simulink model "trajStab"  (R2016b)
settings: Solver=FixedStepAuto  StartTime=0.0  StopTime=12  FixedStep=prms.Ts  RelTol=1e-3
PreLoadFcn:
  | Ts = 1e-3
undefined symbols (not defined in the file or in its folder): DiscIntNeverNeededParam, H, P0, prms, x0
libraries: simulink x1
PreSaveFcn:
  | set_param(gcs, 'location', [15 50 815 560])
settings Model: SimulationMode=external  Creator=The MathWorks Inc.  LastModifiedBy=marti
settings SolverCC: PositivePriorityOrder=on
settings DataIOCC: LimitDataPoints=on  SaveFormat=Array
settings OptimizationCC: BlockReduction=off  BooleanDataType=off  DefaultUnderspecifiedDataType=single  LifeSpan=inf  MaxStackSize=64
settings DebuggingCC: SaveWithParameterizedLinksMsg=none  UnderspecifiedInitializationDetection=Classic  MergeDetectMultiDrivingBlocksExec=none  SignalResolutionControl=TryResolveAllWithWarning  ParameterTunabilityLossMsg=error  SFUnexpectedBacktrackingDiag=warning  SFNoUnconditionalDefaultTransitionDiag=warning  SFExecutionAtInitializationDiag=none
settings HardwareCC: ProdBitPerPointer=32  ProdBitPerSizeT=32  ProdBitPerPtrDiffT=32  ProdLargestAtomicInteger=Long  ProdLargestAtomicFloat=Double  ProdWordSize=32  ProdHWDeviceType=ARM Compatible->ARM Cortex
settings ModelReferenceCC: PropagateSignalLabelsOutOfModel=off
settings RTWCC: SystemTargetFile=ert.tlc  HardwareBoard=Raspberry Pi  TLCOptions=-aInlineSetEventsForThisBaseRateFcn=TLC_FALSE -aSuppressMultiTaskScheduler=TLC_FALSE -aRateBasedStepFcn=0  TemplateMakefile=ert_default_tmf  Description=Embedded Coder  GenerateReport=on  RTWVerbose=off  Toolchain=GNU GCC Raspberry Pi  BuildConfiguration=Specify  IncludeHyperlinkInReport=on  GenerateTraceInfo=on  GenerateTraceReport=on  GenerateTraceReportSl=on  GenerateTraceReportSf=on  GenerateTraceReportEml=on
settings CodeAppCC: ForceParamTrailComments=on  IgnoreCustomStorageClasses=off  OperatorAnnotations=on  SimulinkDataObjDesc=on  SFDataObjDesc=on  MATLABFcnDesc=on  MangleLength=10  InsertBlockDesc=on  MATLABSourceComments=on
settings ERTTargetCC: SupportVariableSizeSignals=on
settings ConfigComp: CovMetricSettings=dw  CovHtmlReporting=on  CovSaveCumulativeToWorkspaceVar=on  CovSaveSingleToWorkspaceVar=on  CovExternalEMLEnable=off  CovSFcnEnable=off

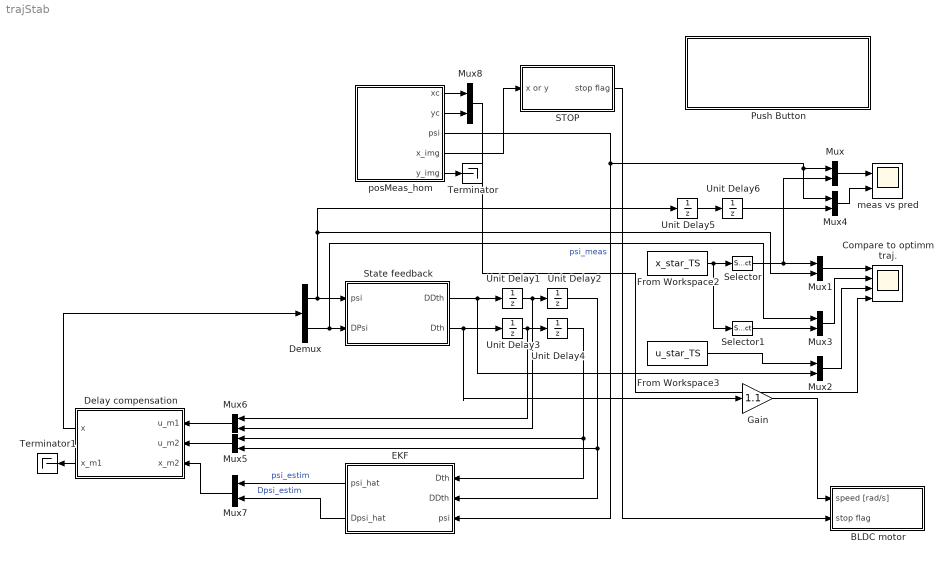
== system trajStab ==
  BLDC motor : Subsystem
  Compare to optimm traj. : Scope  NumInputPorts=4
  Delay compensation : Subsystem
  Demux : Demux  Outputs=2
  EKF : Subsystem
  From Workspace2 : FromWorkspace  VariableName=x_star_TS  OutDataTypeStr=single  SampleTime=prms.Ts  Interpolate=off  OutputAfterFinalValue=Setting to zero
  From Workspace3 : FromWorkspace  VariableName=u_star_TS  SampleTime=prms.Ts  Interpolate=off  OutputAfterFinalValue=Setting to zero
  Gain : Gain  Gain=1.1
  Mux{,1..8} (9 alike) : Mux  Inputs=2
  Push Button : Subsystem  DialogController=hmiCreateDDGDialog  IsWebBlock=on  mask(MWDashboardBlock){webBlockId=aa30e358-d2c6-466c-a89a-de069679829e, webBlockType=pushbutton, ShowInLibBrwoser=on, ShowInitialText=on, HMISrcModelName=trajStab}
      mask prompts: webBlockId "WebBlock Id"; webBlockType "WebBlock Type"; HMISrcModelName "Source Model"
      mask help: SimulinkHMI:dialogs:PushButtonDialogDesc
      mask Help: helpview([docroot '/mapfiles/simulink.map'], 'hmi_push_button')
      mask Display:
      | model = bdroot(gcb);
      | if strcmp(get_param(model,'BlockDiagramType'), 'library')
      |     image([(matlabroot) '/toolbox/simulink/hmi/icons/PushButton.png']);
      | end
  STOP : Subsystem
  Selector : Selector  InputPortWidth=3  IndexOptions=Index vector (dialog)  Indices=2  OutputSizes=1
  Selector1 : Selector  InputPortWidth=3  IndexOptions=Index vector (dialog)  Indices=3  OutputSizes=1
  State feedback : Subsystem
  Terminator : Terminator
  Terminator1 : Terminator
  Unit Delay{1..6} (6 alike) : UnitDelay  SampleTime=-1
  meas vs pred : Scope  NumInputPorts=2
  posMeas_hom : Subsystem
  wires:
  posMeas_hom/3(psi) -> EKF/3(psi), Mux4/1, Mux/1  "psi_meas"
  Mux/1 -> meas vs pred/1
  Mux1/1 -> Compare to optimm traj./1
  From Workspace3/1 -> Mux2/1
  From Workspace2/1 -> Selector1/1, Selector/1
  Selector/1 -> Mux1/1, Mux/2
  State feedback/2(Dth) -> Gain/1, Unit Delay3/1
  Unit Delay1/1 -> Mux6/2, Unit Delay2/1
  Mux5/1 -> Delay compensation/2(u_m2)
  Mux6/1 -> Delay compensation/1(u_m1)
  EKF/2(Dpsi_hat) -> Mux7/2  "Dpsi_estim"
  EKF/1(psi_hat) -> Mux7/1  "psi_estim"
  Unit Delay2/1 -> EKF/2(DDth), Mux5/2
  Unit Delay4/1 -> Mux5/1, EKF/1(Dth)
  Unit Delay3/1 -> Mux6/1, Unit Delay4/1
  Delay compensation/1(x) -> Demux/1
  Demux/2 -> Mux3/1, State feedback/2(DPsi)
  State feedback/1(DDth) -> Unit Delay1/1, Mux2/2
  Demux/1 -> State feedback/1(psi), Mux1/2, Unit Delay5/1
  Mux7/1 -> Delay compensation/3(x_m2)
  Mux3/1 -> Compare to optimm traj./2
  Mux2/1 -> Compare to optimm traj./3
  Selector1/1 -> Mux3/2
  STOP/1(stop flag) -> BLDC motor/2(stop flag)
  Mux4/1 -> meas vs pred/2
  Unit Delay6/1 -> Mux4/2
  Unit Delay5/1 -> Unit Delay6/1
  Delay compensation/2(x_m1) -> Terminator1/1
  posMeas_hom/5(y_img) -> Terminator/1
  posMeas_hom/4(x_img) -> STOP/1(x or y)
  posMeas_hom/1(xc) -> Mux8/1
  posMeas_hom/2(yc) -> Mux8/2
  Mux8/1 -> Compare to optimm traj./4
  Gain/1 -> BLDC motor/1(speed [rad/s])

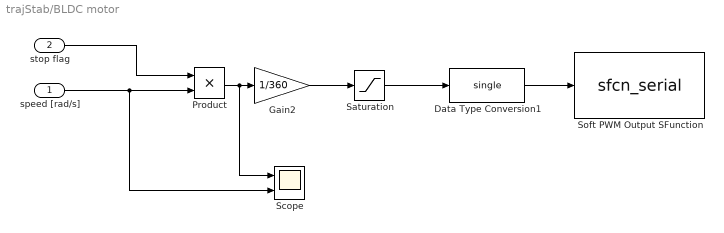
== system trajStab/BLDC motor ==
  speed [rad/s] : Inport
  stop flag : Inport  Port=2
  Data Type Conversion1 : DataTypeConversion  OutDataTypeStr=single
  Gain2 : Gain  Gain=1/360
  Product : Product
  Saturation : Saturate  UpperLimit=0.3  LowerLimit=-0.3
  Scope : Scope  NumInputPorts=2
  Soft PWM Output SFunction : S-Function  InitFcn=try, set_param(gcb,'FunctionName','sfcn_serial'), end  FunctionName=sfcn_serial  SFunctionModules=sfcn_serial_wrapper  SFunctionDeploymentMode=off  EnableBusSupport=off  mask(S-Function Builder){}
      mask init:
      | val = [[.9  0.75 0.75 1 1 .9 .9 1]',[1 1 0.75 0.75 .9 .9 1 .9]'];try , sys = get_param(gcb,'SfunBuilderFcnName');if isempty(sys), sys = get_param(gcb,'FunctionName'); end,catch, sys = get_param(gcb,'FunctionName'); end
      settings: CopyFcn=set_param(gcbh,'LinkStatus','none')  PreSaveFcn=try, set_param(gcb,'FunctionName','sfcn_serial'), end  OpenFcn=sfunctionwizard(gcbh)
      mask Display: plot(val(:,1),val(:,2)),disp(sys), port_label('input',1,'in')
  wires:
  Saturation/1 -> Data Type Conversion1/1
  Gain2/1 -> Saturation/1
  Data Type Conversion1/1 -> Soft PWM Output SFunction/1
  Product/1 -> Scope/1, Gain2/1
  speed [rad/s]/1 -> Scope/2, Product/2
  stop flag/1 -> Product/1

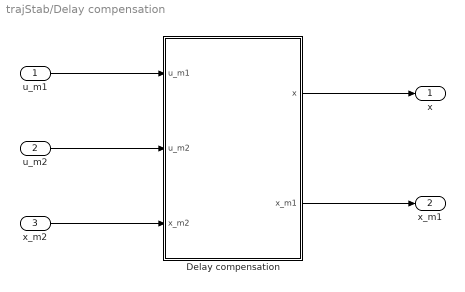
== system trajStab/Delay compensation ==
  u_m1 : Inport
  u_m2 : Inport  Port=2
  x_m2 : Inport  Port=3
  Delay compensation : MATLAB Function  TreatAsAtomicUnit=on  SystemSampleTime=prms.Ts
  x : Outport
  x_m1 : Outport  Port=2
  wires:
  x_m2/1 -> Delay compensation/3(x_m2)
  u_m1/1 -> Delay compensation/1(u_m1)
  u_m2/1 -> Delay compensation/2(u_m2)
  Delay compensation/1(x) -> x/1
  Delay compensation/2(x_m1) -> x_m1/1

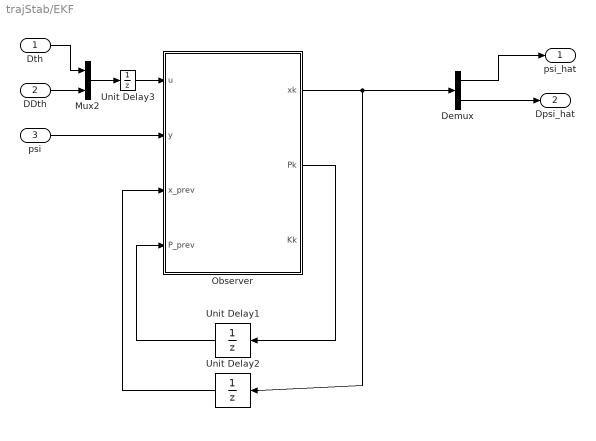
== system trajStab/EKF ==
  Dth : Inport
  DDth : Inport  Port=2
  psi : Inport  Port=3
  Demux : Demux  Outputs=2
  Mux2 : Mux  Inputs=2
  Observer : MATLAB Function  TreatAsAtomicUnit=on  SystemSampleTime=prms.Ts
  Unit Delay1 : UnitDelay  InitialCondition=P0  SampleTime=-1
  Unit Delay2 : UnitDelay  InitialCondition=x0  SampleTime=-1
  Unit Delay3 : UnitDelay  SampleTime=-1
  psi_hat : Outport
  Dpsi_hat : Outport  Port=2
  wires:
  Unit Delay2/1 -> Observer/3(x_prev)
  Observer/2(Pk) -> Unit Delay1/1
  Unit Delay1/1 -> Observer/4(P_prev)
  Observer/1(xk) -> Demux/1, Unit Delay2/1
  Demux/2 -> Dpsi_hat/1
  Demux/1 -> psi_hat/1
  Mux2/1 -> Unit Delay3/1
  Dth/1 -> Mux2/1
  DDth/1 -> Mux2/2
  psi/1 -> Observer/2(y)
  Unit Delay3/1 -> Observer/1(u)

== system trajStab/Push Button ==

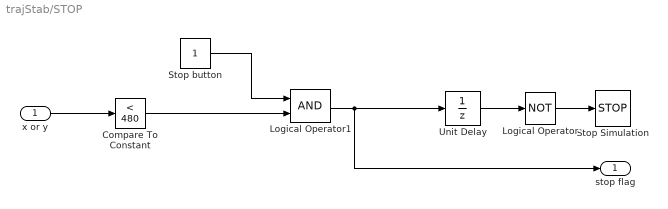
== system trajStab/STOP ==
  x or y : Inport
  Compare To Constant : simulink/Logic and Bit Operations/Compare To Constant  relop=<  const=480  OutDataTypeStr=boolean
  Logical Operator : Logic  Operator=NOT  AllPortsSameDT=off  OutDataTypeStr=boolean
  Logical Operator1 : Logic  AllPortsSameDT=off  OutDataTypeStr=boolean
  Stop Simulation : Stop
  Stop button : Constant
  Unit Delay : UnitDelay  InitialCondition=1  SampleTime=-1
  stop flag : Outport
  wires:
  Logical Operator/1 -> Stop Simulation/1
  Logical Operator1/1 -> stop flag/1, Unit Delay/1
  Unit Delay/1 -> Logical Operator/1
  Compare To Constant/1 -> Logical Operator1/2
  Stop button/1 -> Logical Operator1/1
  x or y/1 -> Compare To Constant/1

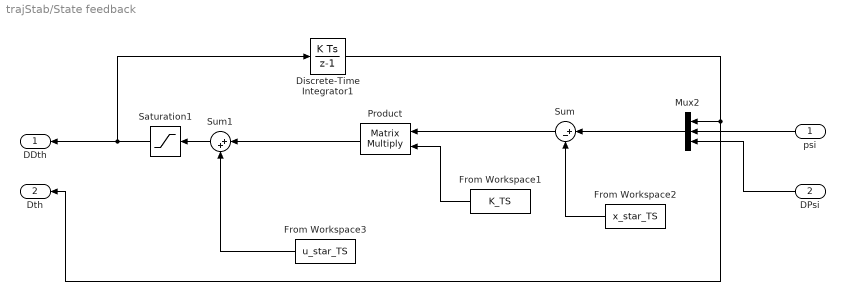
== system trajStab/State feedback ==
  psi : Inport
  DPsi : Inport  Port=2
  Discrete-Time Integrator1 : DiscreteIntegrator  InitialConditionSetting=State (most efficient)  SampleTime=prms.Ts  ICPrevOutput=DiscIntNeverNeededParam  ICPrevScaledInput=DiscIntNeverNeededParam
  From Workspace1 : FromWorkspace  VariableName=K_TS  OutDataTypeStr=single  SampleTime=prms.Ts  Interpolate=off  OutputAfterFinalValue=Setting to zero
  From Workspace2 : FromWorkspace  VariableName=x_star_TS  OutDataTypeStr=single  SampleTime=prms.Ts  Interpolate=off  OutputAfterFinalValue=Setting to zero
  From Workspace3 : FromWorkspace  VariableName=u_star_TS  OutDataTypeStr=single  SampleTime=prms.Ts  Interpolate=off  OutputAfterFinalValue=Setting to zero
  Mux2 : Mux  Inputs=3
  Product : Product  Multiplication=Matrix(*)
  Saturation1 : Saturate  UpperLimit=prms.usat  LowerLimit=-prms.usat
  Sum : Sum  Inputs=|+-
  Sum1 : Sum  Inputs=|++
  DDth : Outport
  Dth : Outport  Port=2
  wires:
  From Workspace1/1 -> Product/2
  Mux2/1 -> Sum/1
  From Workspace2/1 -> Sum/2
  Sum/1 -> Product/1
  From Workspace3/1 -> Sum1/2
  Sum1/1 -> Saturation1/1
  Saturation1/1 -> Discrete-Time Integrator1/1, DDth/1
  Discrete-Time Integrator1/1 -> Dth/1, Mux2/1
  psi/1 -> Mux2/2
  DPsi/1 -> Mux2/3
  Product/1 -> Sum1/1

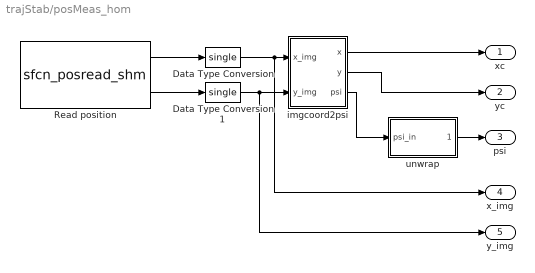
== system trajStab/posMeas_hom ==
  Data Type Conversion : DataTypeConversion  OutDataTypeStr=single
  Data Type Conversion1 : DataTypeConversion  OutDataTypeStr=single
  Read position : S-Function  InitFcn=try, set_param(gcb,'FunctionName','sfcn_posread_shm'), end  FunctionName=sfcn_posread_shm  SFunctionModules=sfcn_posread_shm_wrapper  SFunctionDeploymentMode=off  EnableBusSupport=off  mask(S-Function Builder){}
      mask init: same as trajStab/BLDC motor/Soft PWM Output SFunction
      settings: CopyFcn=set_param(gcbh,'LinkStatus','none')  PreSaveFcn=try, set_param(gcb,'FunctionName','sfcn_posread_shm'), end  OpenFcn=sfunctionwizard(gcbh)
      mask Display: plot(val(:,1),val(:,2)),disp(sys), port_label('output',1,'pos_x'), port_label('output',2,'pos_y')
  imgcoord2psi : Subsystem
  unwrap : Subsystem
  xc : Outport
  yc : Outport  Port=2
  psi : Outport  Port=3
  x_img : Outport  Port=4
  y_img : Outport  Port=5
  wires:
  Read position/1 -> Data Type Conversion/1
  Data Type Conversion/1 -> x_img/1, imgcoord2psi/1(x_img)
  Data Type Conversion1/1 -> y_img/1, imgcoord2psi/2(y_img)
  Read position/2 -> Data Type Conversion1/1
  imgcoord2psi/3(psi) -> unwrap/1(psi_in)
  unwrap/1(psi_out) -> psi/1
  imgcoord2psi/1(x) -> xc/1
  imgcoord2psi/2(y) -> yc/1

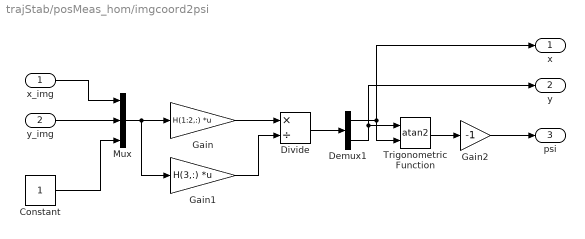
== system trajStab/posMeas_hom/imgcoord2psi ==
  x_img : Inport
  y_img : Inport  Port=2
  Constant : Constant  OutDataTypeStr=single
  Demux1 : Demux  Outputs=2
  Divide : Product  Inputs=*/
  Gain : Gain  Gain=H(1:2,:)  Multiplication=Matrix(K*u)
  Gain1 : Gain  Gain=H(3,:)  Multiplication=Matrix(K*u)
  Gain2 : Gain  Gain=-1  OutDataTypeStr=single
  Mux : Mux  Inputs=3
  Trigonometric Function : Trigonometry  Operator=atan2  OutputSignalType=real
  x : Outport
  y : Outport  Port=2
  psi : Outport  Port=3
  wires:
  Mux/1 -> Gain1/1, Gain/1
  Constant/1 -> Mux/3
  Demux1/2 -> y/1, Trigonometric Function/1
  Gain/1 -> Divide/1
  Gain1/1 -> Divide/2
  Divide/1 -> Demux1/1
  Demux1/1 -> x/1, Trigonometric Function/2
  x_img/1 -> Mux/1
  y_img/1 -> Mux/2
  Trigonometric Function/1 -> Gain2/1
  Gain2/1 -> psi/1

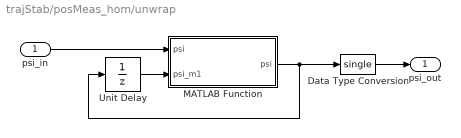
== system trajStab/posMeas_hom/unwrap ==
  psi_in : Inport
  Data Type Conversion : DataTypeConversion  OutDataTypeStr=single
  MATLAB Function : MATLAB Function  TreatAsAtomicUnit=on
  Unit Delay : UnitDelay  InitialCondition=single(0)  SampleTime=-1
  psi_out : Outport
  wires:
  MATLAB Function/1(psi) -> Data Type Conversion/1, Unit Delay/1
  Unit Delay/1 -> MATLAB Function/2(psi_m1)
  psi_in/1 -> MATLAB Function/1("psi ")
  Data Type Conversion/1 -> psi_out/1

== matlab function trajStab/Delay compensation/Delay compensation ==
  data: u_m1 input; u_m2 input; x output; x_m2 input; prms parameter; x_m1 output
function [x, x_m1] = delayCompensation( u_m1, u_m2, x_m2, prms)

a =  prms.out.a_bar;
b =  prms.out.b_bar;
c =  prms.out.c_bar;
d =  prms.out.d_bar;
e =  prms.out.e_bar;

N = 1;
T = prms.Ts/N;

% Time Update - 1
x_old = x_m2;
x_new = single([0; 0]);
for i = 1:N
    x_new(1) = x_old(1) + T*x_old(2);
    x_new(2) = x_old(2) + T* 1/a*(-c*sin(x_old(1)) - b*x_old(2) - d*u_m2(1) + e*u_m2(2));    
    x_old = x_new;
end
x_m1 = x_new;

% Time Update - 2
x_old = x_m1;
x_new = single([0; 0]);
for i = 1:N
    x_new(1) = x_old(1) + T*x_old(2);
    x_new(2) = x_old(2) + T*1/a*(-c*sin(x_old(1)) - b*x_old(2) - d*u_m1(1) + e*u_m1(2));    
    x_old = x_new;
end
x = x_new;

== matlab function trajStab/EKF/Observer ==
  data: u input; y input; xk output single; x_prev input; P_prev input; Pk output; Kk output; prms parameter
function [xk, Pk, Kk] = EKF( u, y, x_prev, P_prev, prms)

a =  prms.out.a_bar;
b =  prms.out.b_bar;
c =  prms.out.c_bar;
d =  prms.out.d_bar;
e =  prms.out.e_bar;

Q =  prms.out.KF.Q;
R =  prms.out.KF.R;

Ak_c = [0 1; -c/a*cos(x_prev(1)) -b/a]; % system matrix of the linearized continuous model
Ak = eye(2) + prms.Ts*Ak_c; % discretized version of the system matrix
Hk = [1 0];

% Time Update
xk = single([0; 0]);
xk(1) = x_prev(1) + prms.Ts*x_prev(2);
xk(2) = x_prev(2) + prms.Ts * 1/a*(-c*sin(x_prev(1)) - b*x_prev(2) - d*u(1) + e*u(2));
% xk = Ak*x_prev + Bk*u;
Pk = Ak*P_prev*Ak'+Q;

% Measurement Update
Kk = Pk*Hk'/(Hk*Pk*Hk'+R);
xk = xk + Kk*(y-Hk*xk);
Pk = (eye(2)-Kk*Hk)*Pk;

== matlab function trajStab/posMeas_hom/unwrap/MATLAB Function ==
  data: psi input; psi output; psi_m1 input
function psi = unwrap(psi, psi_m1)
%%% The code is taken from the Matlab function unwrap

% Unwrap phase angles.  Algorithm minimizes the incremental phase variation 
% by constraining it to the range [-pi,pi]
dp = psi - psi_m1;                % Incremental phase variations

% Compute an integer describing how many times 2*pi we are off:
% dp in [-pi, pi]: dp_corr = 0,
% elseif dp in [-3*pi, 3*pi]: dp_corr = 1,
% else if dp in [-5*pi, 5*pi]: dp_corr = 2, ...
dp_corr = dp./(2*pi);

% We want to do round(dp_corr), except that we want the tie-break at n+0.5
% to round towards zero instead of away from zero (that is, (2n+1)*pi will
% be shifted by 2n*pi, not by (2n+2)*pi):
roundDown = abs(rem(dp_corr, 1)) <= 0.5;
dp_corr(roundDown) = fix(dp_corr(roundDown));

dp_corr = round(dp_corr);

% Stop the jump from happening if dp < cutoff (no effect if cutoff <= pi)
dp_corr(abs(dp) < pi) = 0;

% Integrate corrections and add to P to produce smoothed phase values
psi = single(psi - (2*pi)*cumsum(dp_corr,1));
